simulink model "5_pole_simulink"  (R2023b)
settings: Solver=VariableStepAuto  StartTime=0.0  StopTime=20  RelTol=1e-3
settings Model: Creator=mampane  LastModifiedBy=dkim4

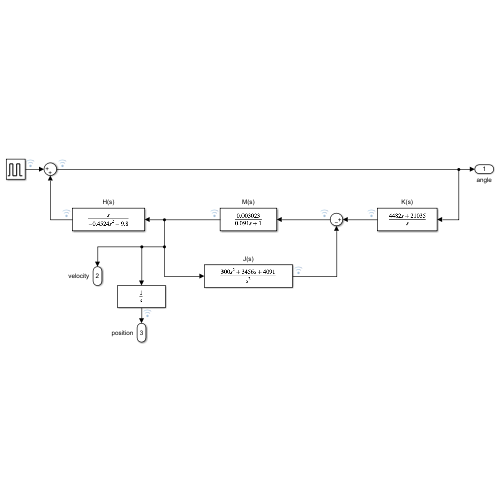
[thumbnail: Simulink's stored preview of the top-level diagram]
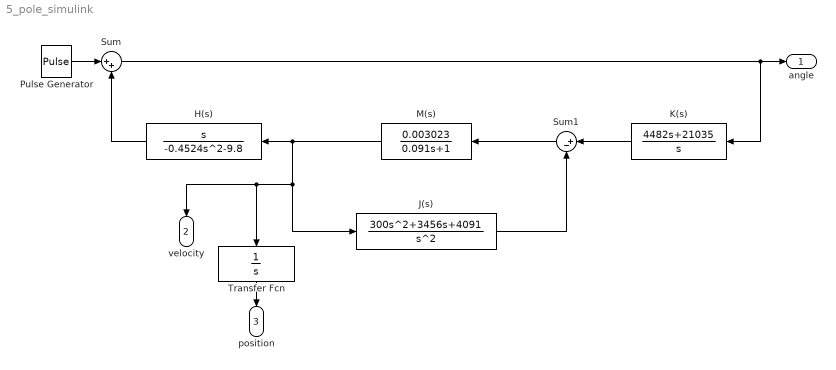
== system 5_pole_simulink ==
  H(s) : TransferFcn  Numerator=[1 0]  Denominator=[-0.4524 0 -9.8]
  J(s) : TransferFcn  Numerator=[300 3456 4091]  Denominator=[1 0 0]
  K(s) : TransferFcn  Numerator=[4482 21035]  Denominator=[1 0]
  M(s) : TransferFcn  Numerator=[0.003023]  Denominator=[0.091 1]
  Pulse Generator : DiscretePulseGenerator  PulseType=Time based  Amplitude=1/36  Period=10  PulseWidth=0.1
  Sum : Sum  Inputs=|++
  Sum1 : Sum  Inputs=|+-
  Transfer Fcn : TransferFcn  Denominator=[1 0]
  angle : Outport
  velocity : Outport  Port=2
  position : Outport  Port=3
  wires:
  Pulse Generator/1 -> Sum/1
  Sum/1 -> angle/1, K(s)/1
  K(s)/1 -> Sum1/1
  Sum1/1 -> M(s)/1
  M(s)/1 -> velocity/1, Transfer Fcn/1, J(s)/1, H(s)/1
  H(s)/1 -> Sum/2
  J(s)/1 -> Sum1/2
  Transfer Fcn/1 -> position/1
